simulink model "cascade7"  (R2020a)
settings: Solver=VariableStepAuto  StartTime=0.0  StopTime=10.0  RelTol=1e-3
libraries: simulink x1
settings Model: Creator=I3  LastModifiedBy=I3

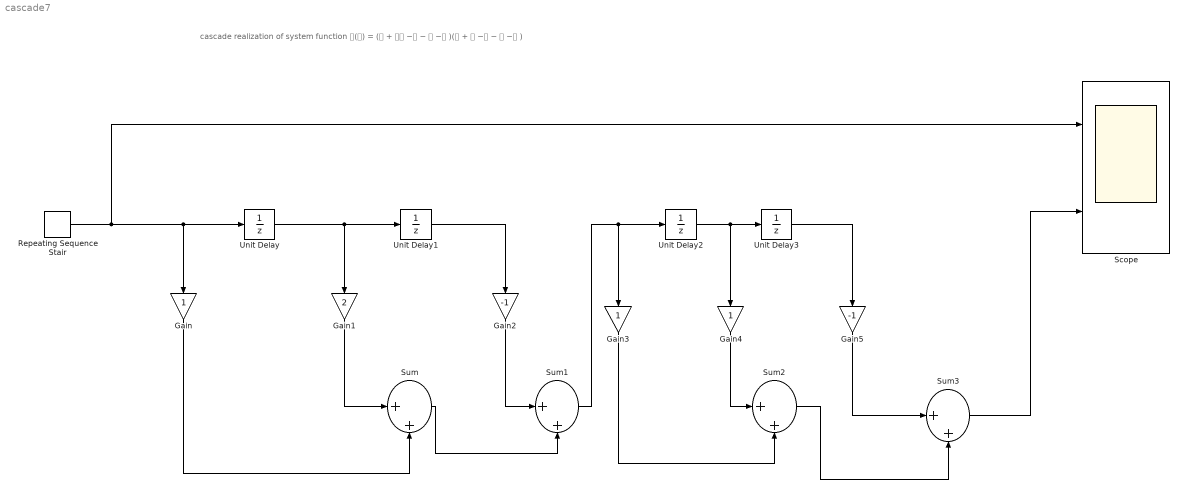
== system cascade7 ==
  note: cascade realization of system function 𝐇(𝐳) = (𝟏 + 𝟐𝐳 −𝟏 − 𝐳 −𝟐 )(𝟏 + 𝐳 −𝟏 − 𝐳 −𝟐 )
  Gain : Gain
  Gain1 : Gain  Gain=2
  Gain2 : Gain  Gain=-1
  Gain3 : Gain
  Gain4 : Gain
  Gain5 : Gain  Gain=-1
  Repeating Sequence Stair : simulink/Sources/Repeating Sequence Stair  OutValues=[1 0 1 0 1 0 0 0 0 0 1 1].'  tsamp=-1  OutMin=[]  OutMax=[]  OutDataTypeStr=double  OutputDataTypeScalingMode=double  OutDataType=fixdt(0,8)  ConRadixGroup=Best Precision: Vector-wise  OutScaling=2^-12
  Scope : Scope  NumInputPorts=2
  Sum{,1..3} (4 alike) : Sum  Inputs=|++
  Unit Delay{,1..3} (4 alike) : UnitDelay  SampleTime=-1  HasFrameUpgradeWarning=on
  wires:
  Repeating Sequence Stair/1 -> Scope/1, Gain/1, Unit Delay/1
  Unit Delay/1 -> Gain1/1, Unit Delay1/1
  Unit Delay2/1 -> Gain4/1, Unit Delay3/1
  Unit Delay3/1 -> Gain5/1
  Unit Delay1/1 -> Gain2/1
  Sum1/1 -> Unit Delay2/1, Gain3/1
  Gain3/1 -> Sum2/2
  Gain4/1 -> Sum2/1
  Gain5/1 -> Sum3/1
  Sum3/1 -> Scope/2
  Gain/1 -> Sum/2
  Gain1/1 -> Sum/1
  Sum/1 -> Sum1/2
  Gain2/1 -> Sum1/1
  Sum2/1 -> Sum3/2
